simulink model "PCM"  (Simulink 8.2)
settings: Solver=ode45  StartTime=0.0  StopTime=10.0  FixedStep=1/10000  RelTol=1e-3
libraries: commutil2 x2, commchan3 x1
settings Model: Creator=Yi_Liu  LastModifiedBy=Yi_Liu
settings DataIOCC: SignalLoggingSaveFormat=Dataset
settings OptimizationCC: ExpressionDepthLimit=128
settings DebuggingCC: FcnCallInpInsideContextMsg=EnableAllAsError  StateNameClashWarn=none
settings GRTTargetCC: CombineOutputUpdateFcns=on  GRTInterface=off

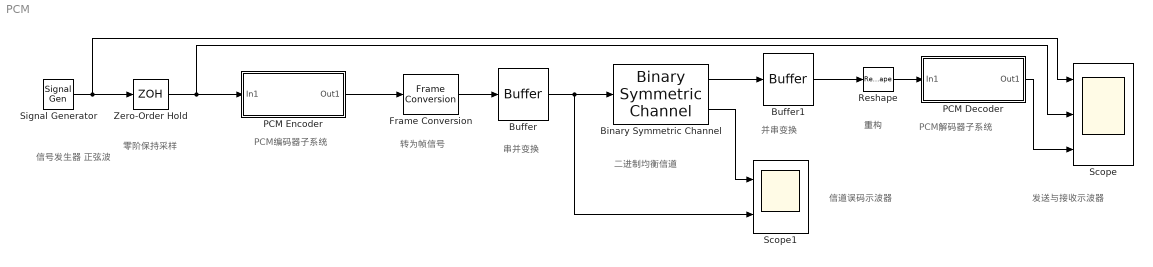
== system PCM ==
  note: 发送与接收示波器
  note: 信道误码示波器
  note: PCM解码器子系统
  note: 重构
  note: 并串变换
  note: 二进制均衡信道
  note: 串并变换
  note: 转为帧信号
  note: PCM编码器子系统
  note: 零阶保持采样
  note: 信号发生器
      | 正弦波
  Binary Symmetric Channel : commchan3/Binary Symmetric Channel  P=0.01  s=64  E=on  outDtype=double
  Buffer : Buffer  N=1  TreatMby1Signals=One channel
  Buffer1 : Buffer  N=8  TreatMby1Signals=One channel
  Frame Conversion : FrameConversion
  PCM Decoder : Subsystem
  PCM Encoder : Subsystem
  Reshape : Reshape
  Scope : Scope  NumInputPorts=3
      settings: YMin=-5~-5~-2  YMax=5~5~2
  Scope1 : Scope  NumInputPorts=2
      settings: YMin=-5~-5  YMax=5~5
  Signal Generator : SignalGenerator  Frequency=200
  Zero-Order Hold : ZeroOrderHold  SampleTime=1/16000
  wires:
  Frame Conversion/1 -> Buffer/1
  Buffer1/1 -> Reshape/1
  Reshape/1 -> PCM Decoder/1(In1)
  Binary Symmetric Channel/1 -> Buffer1/1
  Buffer/1 -> Scope1/2, Binary Symmetric Channel/1
  Binary Symmetric Channel/2 -> Scope1/1
  Signal Generator/1 -> Scope/1, Zero-Order Hold/1
  Zero-Order Hold/1 -> Scope/2, PCM Encoder/1(In1)
  PCM Encoder/1(Out1) -> Frame Conversion/1
  PCM Decoder/1(Out1) -> Scope/3

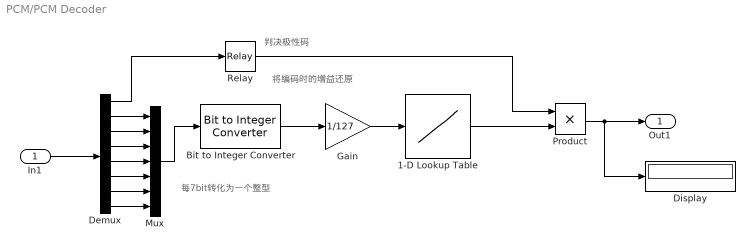
== system PCM/PCM Decoder ==
  note: 判决极性码
  note: 将编码时的增益还原
  note: 每7bit转化为一个整型
  In1 : Inport
  1-D Lookup Table : Lookup_n-D  NumberOfTableDimensions=1  BreakpointsForDimension1=[-5:5]  Table=tanh([-5:5])  InternalRulePriority=Speed  RndMeth=Simplest  InputSameDT=on
  Bit to Integer Converter : commutil2/Bit to Integer Converter  nbits=7  bitOrder=MSB first  signedOutputValues=Unsigned  outDtype=Inherit via internal rule  outDtypeSigned=Inherit via internal rule
  Demux : Demux  Outputs=8
  Display : Display
  Gain : Gain  Gain=1/127
  Mux : Mux  Inputs=7
  Product : Product
  Relay : Relay  OffOutputValue=-1
  Out1 : Outport
  wires:
  In1/1 -> Demux/1
  Bit to Integer Converter/1 -> Gain/1
  Gain/1 -> 1-D Lookup Table/1
  1-D Lookup Table/1 -> Product/2
  Relay/1 -> Product/1
  Product/1 -> Display/1, Out1/1
  Mux/1 -> Bit to Integer Converter/1
  Demux/1 -> Relay/1
  Demux/2 -> Mux/1
  Demux/3 -> Mux/2
  Demux/4 -> Mux/3
  Demux/5 -> Mux/4
  Demux/6 -> Mux/5
  Demux/7 -> Mux/6
  Demux/8 -> Mux/7

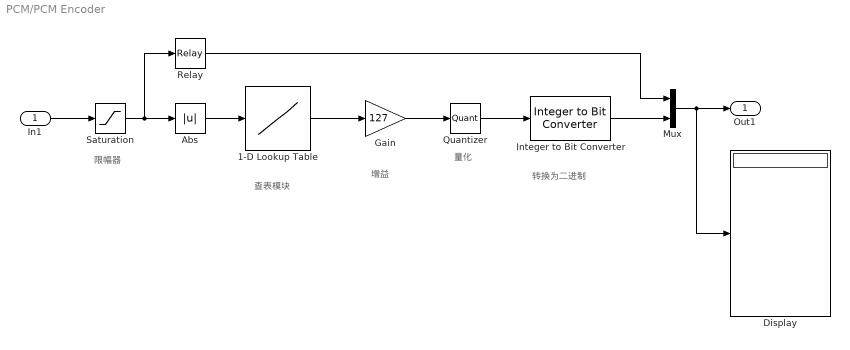
== system PCM/PCM Encoder ==
  note: 量化
  note: 转换为二进制
  note: 增益
  note: 查表模块
  note: 限幅器
  In1 : Inport
  1-D Lookup Table : Lookup_n-D  NumberOfTableDimensions=1  BreakpointsForDimension1=[-5:5]  Table=tanh([-5:5])  InternalRulePriority=Speed  RndMeth=Simplest  InputSameDT=on
  Abs : Abs
  Display : Display
  Gain : Gain  Gain=127
  Integer to Bit Converter : commutil2/Integer to Bit Converter  nbits=7  signedInputValues=Unsigned  bitOrder=MSB first  outDtype=Inherit via internal rule
  Mux : Mux  Inputs=2
  Quantizer : Quantizer  QuantizationInterval=1
  Relay : Relay
  Saturation : Saturate  UpperLimit=1  LowerLimit=-1
  Out1 : Outport
  wires:
  In1/1 -> Saturation/1
  Saturation/1 -> Relay/1, Abs/1
  Abs/1 -> 1-D Lookup Table/1
  1-D Lookup Table/1 -> Gain/1
  Gain/1 -> Quantizer/1
  Quantizer/1 -> Integer to Bit Converter/1
  Integer to Bit Converter/1 -> Mux/2
  Mux/1 -> Display/1, Out1/1
  Relay/1 -> Mux/1
